simulink model "Matematico_Modelo_final"  (R2022b)
settings: Solver=VariableStepAuto  StartTime=0.0  StopTime=200  RelTol=1e-3
values from neighbouring files (symbols this model uses):
  B = 0.0244    [Datos_motor.m]
  Ff = 0.74    [Datos_motor.m]
  G = 50    [Datos_motor.m]
  J1 = 0.00072    [Datos_motor.m]
  J2 = 0.00072    [Datos_motor.m]
  Jg = 9.158    [Datos_motor.m]
  Jm = 9.158    [Datos_motor.m]
  K1 = 7.23e10    (= 72300000000)    [Datos_motor.m]
  K2 = 7.23e10    (= 72300000000)    [Datos_motor.m]
  K3 = 7.23e10    (= 72300000000)    [Datos_motor.m]
  Ke = 0.623    [Datos_motor.m]
  Kt = 0.333    [Datos_motor.m]
  L = 0.00163    [Datos_motor.m]
  Mcx = 1.1414    [Datos_motor.m]
  Mcy = 2.036    [Datos_motor.m]
  McZ = 0.839    [Datos_motor.m]
  R = 2.1    [Datos_motor.m]
  T = 2.059    [Datos_motor.m]
libraries: slpidlib x3
settings Model: Creator=aleal  LastModifiedBy=USER
settings DebuggingCC: UnconnectedInputMsg=warning  UnconnectedOutputMsg=warning  UnconnectedLineMsg=warning
settings ModelReferenceCC: EnableRefExpFcnMdlSchedulingChecks=on
settings RTWCC: DLArmComputeVersion=19.05

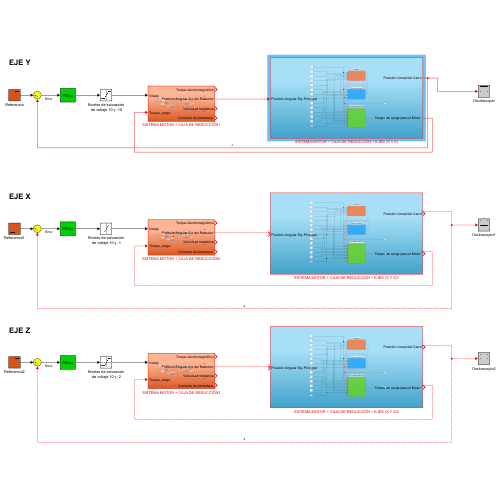
[thumbnail: Simulink's stored preview of the top-level diagram]
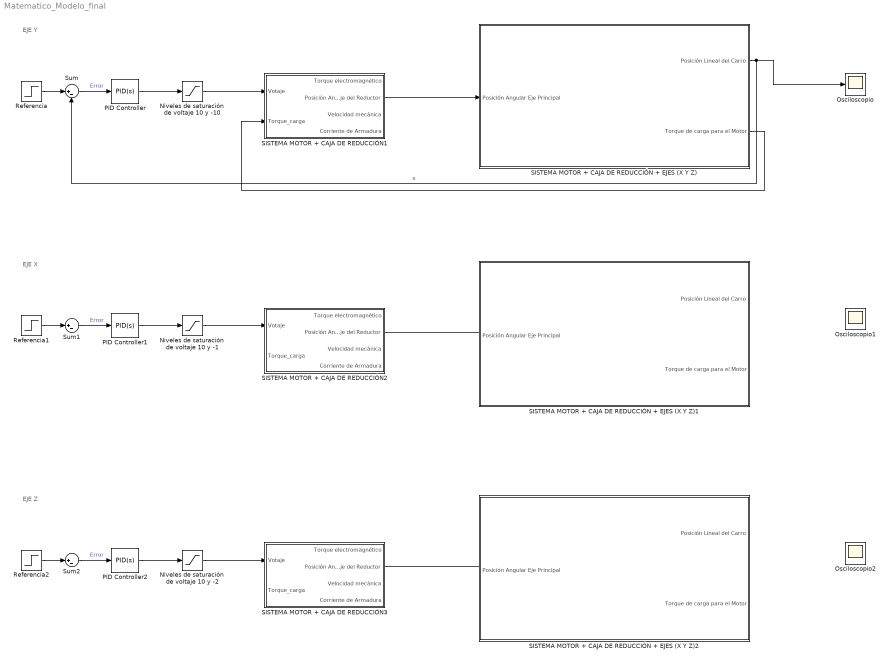
== system Matematico_Modelo_final ==
  note: EJE Z
  note: EJE Y
  note: EJE X
  Niveles de saturación de voltaje 10 y -1 : Saturate  UpperLimit=10  LowerLimit=-10
  Niveles de saturación de voltaje 10 y -10 : Saturate  UpperLimit=10  LowerLimit=-10
  Niveles de saturación de voltaje 10 y -2 : Saturate  UpperLimit=10  LowerLimit=-10
  Osciloscopio : Scope
  Osciloscopio1 : Scope
  Osciloscopio2 : Scope
  PID Controller : slpidlib/PID Controller  Controller=PID  Form=Parallel  TimeDomain=Continuous-time  UseExternalTs=off  SampleTime=-1  IntegratorMethod=Forward Euler  FilterMethod=Forward Euler  ControllerParametersSource=internal  P=10.0  I=1.0  UseKiTs=off  D=1.3  N=100  UseFilter=on  TunerSelectOption=Transfer Function Based (PID Tuner App)  InitialConditionSource=internal  InitialConditionForIntegrator=0  InitialConditionForFilter=0  DifferentiatorICPrevScaledInput=0  ExternalReset=none  TrackingMode=off  Kt=1  LimitOutput=off  SatLimitsSource=internal  UpperSaturationLimit=inf  LowerSaturationLimit=-inf  LinearizeAsGain=on  AntiWindupMode=none  Kb=1  LimitIntegrator=off  UpperIntegratorSaturationLimit=inf  LowerIntegratorSaturationLimit=-inf  POutMin=[]  POutMax=[]  IOutMin=[]  IOutMax=[]  DOutMin=[]  DOutMax=[]  NOutMin=[]  NOutMax=[]  SumOutMin=[]  SumOutMax=[]  SaturationOutMin=[]  SaturationOutMax=[]  PParamMin=[]  PParamMax=[]  IParamMin=[]  IParamMax=[]  DParamMin=[]  DParamMax=[]  NParamMin=[]  NParamMax=[]  KbParamMin=[]  KbParamMax=[]  KtParamMin=[]  KtParamMax=[]  KbOutMin=[]  KbOutMax=[]  KtOutMin=[]  KtOutMax=[]  IntegratorOutMin=[]  IntegratorOutMax=[]  FilterOutMin=[]  FilterOutMax=[]  SumI1OutMin=[]  SumI1OutMax=[]  SumI2OutMin=[]  SumI2OutMax=[]  SumI3OutMin=[]  SumI3OutMax=[]  SumI4OutMin=[]  SumI4OutMax=[]  SumDOutMin=[]  SumDOutMax=[]  DifferentiatorOutMin=[]  DifferentiatorOutMax=[]  FilterDiffOutCoefMin=[]  FilterDiffOutCoefMax=[]  ReciprocalOutMin=[]  ReciprocalOutMax=[]  SumDenOutMin=[]  SumDenOutMax=[]  SumNumOutMin=[]  SumNumOutMax=[]  DivideOutMin=[]  DivideOutMax=[]  UdiffTsProdOutMin=[]  UdiffTsProdOutMax=[]  NTsProdOutMin=[]  NTsProdOutMax=[]  UintegralTsProdOutMin=[]  UintegralTsProdOutMax=[]  UngainTsProdOutMin=[]  UngainTsProdOutMax=[]  ClampingZeroOutDataTypeStr=Inherit: Inherit via back propagation  ClampingZeroOutMin=[]  ClampingZeroOutMax=[]  FilterDenConstantOutDataTypeStr=Inherit: Inherit via back propagation  FilterDenConstantOutMin=[]  FilterDenConstantOutMax=[]  PCopyOutDataTypeStr=Inherit: Inherit via back propagation  PCopyOutMin=[]  PCopyOutMax=[]  NCopyOutDataTypeStr=Inherit: Inherit via back propagation  NCopyOutMin=[]  NCopyOutMax=[]  IntegratorContinuousStateAttributes=''  IntegratorStateMustResolveToSignalObject=off  IntegratorRTWStateStorageClass=Auto  FilterContinuousStateAttributes=''  FilterStateMustResolveToSignalObject=off  FilterRTWStateStorageClass=Auto  ParallelPVariant=InternalParameters  IdealPVariant=Disabled  IVariant=InternalParameters  DVariant=InternalParameters  IntegratorVariant=Continuous  SatVariant=Disabled  AWVariant=Passthrough  PCopyVariant=Disabled  TRVariant=Disabled  FdbkBlocksVariant=Forward  IdealPFdbkVariant=Disabled  SatFdbkVariant=Disabled  DerivativeFilterVariant=ContFilter  NVariant=InternalParameters  NCopyVariant=Disabled  FilterICVariant=InternalICsFilter  IntegratorICVariant=InternalICs  ExternalResetVariant=Disabled  TRSumVariant=Passthrough  SumFdbkVariant=Disabled  SumVariant=Sum_PID  TsampFilterVariant=InternalTs  TsampNgainVariant=Passthrough  TsampIntegralVariant=Passthrough  ExternalSaturationOutDataTypeStr=Inherit: Same as second input
  PID Controller1 : slpidlib/PID Controller  Controller=PID  Form=Parallel  TimeDomain=Continuous-time  UseExternalTs=off  SampleTime=-1  IntegratorMethod=Forward Euler  FilterMethod=Forward Euler  ControllerParametersSource=internal  P=9.0  I=0.7  UseKiTs=off  D=0.8  N=100  UseFilter=on  TunerSelectOption=Transfer Function Based (PID Tuner App)  InitialConditionSource=internal  InitialConditionForIntegrator=0  InitialConditionForFilter=0  DifferentiatorICPrevScaledInput=0  ExternalReset=none  TrackingMode=off  Kt=1  LimitOutput=off  SatLimitsSource=internal  UpperSaturationLimit=inf  LowerSaturationLimit=-inf  LinearizeAsGain=on  AntiWindupMode=none  Kb=1  LimitIntegrator=off  UpperIntegratorSaturationLimit=inf  LowerIntegratorSaturationLimit=-inf  POutMin=[]  POutMax=[]  IOutMin=[]  IOutMax=[]  DOutMin=[]  DOutMax=[]  NOutMin=[]  NOutMax=[]  SumOutMin=[]  SumOutMax=[]  SaturationOutMin=[]  SaturationOutMax=[]  PParamMin=[]  PParamMax=[]  IParamMin=[]  IParamMax=[]  DParamMin=[]  DParamMax=[]  NParamMin=[]  NParamMax=[]  KbParamMin=[]  KbParamMax=[]  KtParamMin=[]  KtParamMax=[]  KbOutMin=[]  KbOutMax=[]  KtOutMin=[]  KtOutMax=[]  IntegratorOutMin=[]  IntegratorOutMax=[]  FilterOutMin=[]  FilterOutMax=[]  SumI1OutMin=[]  SumI1OutMax=[]  SumI2OutMin=[]  SumI2OutMax=[]  SumI3OutMin=[]  SumI3OutMax=[]  SumI4OutMin=[]  SumI4OutMax=[]  SumDOutMin=[]  SumDOutMax=[]  DifferentiatorOutMin=[]  DifferentiatorOutMax=[]  FilterDiffOutCoefMin=[]  FilterDiffOutCoefMax=[]  ReciprocalOutMin=[]  ReciprocalOutMax=[]  SumDenOutMin=[]  SumDenOutMax=[]  SumNumOutMin=[]  SumNumOutMax=[]  DivideOutMin=[]  DivideOutMax=[]  UdiffTsProdOutMin=[]  UdiffTsProdOutMax=[]  NTsProdOutMin=[]  NTsProdOutMax=[]  UintegralTsProdOutMin=[]  UintegralTsProdOutMax=[]  UngainTsProdOutMin=[]  UngainTsProdOutMax=[]  ClampingZeroOutDataTypeStr=Inherit: Inherit via back propagation  ClampingZeroOutMin=[]  ClampingZeroOutMax=[]  FilterDenConstantOutDataTypeStr=Inherit: Inherit via back propagation  FilterDenConstantOutMin=[]  FilterDenConstantOutMax=[]  PCopyOutDataTypeStr=Inherit: Inherit via back propagation  PCopyOutMin=[]  PCopyOutMax=[]  NCopyOutDataTypeStr=Inherit: Inherit via back propagation  NCopyOutMin=[]  NCopyOutMax=[]  IntegratorContinuousStateAttributes=''  IntegratorStateMustResolveToSignalObject=off  IntegratorRTWStateStorageClass=Auto  FilterContinuousStateAttributes=''  FilterStateMustResolveToSignalObject=off  FilterRTWStateStorageClass=Auto  ParallelPVariant=InternalParameters  IdealPVariant=Disabled  IVariant=InternalParameters  DVariant=InternalParameters  IntegratorVariant=Continuous  SatVariant=Disabled  AWVariant=Passthrough  PCopyVariant=Disabled  TRVariant=Disabled  FdbkBlocksVariant=Forward  IdealPFdbkVariant=Disabled  SatFdbkVariant=Disabled  DerivativeFilterVariant=ContFilter  NVariant=InternalParameters  NCopyVariant=Disabled  FilterICVariant=InternalICsFilter  IntegratorICVariant=InternalICs  ExternalResetVariant=Disabled  TRSumVariant=Passthrough  SumFdbkVariant=Disabled  SumVariant=Sum_PID  TsampFilterVariant=InternalTs  TsampNgainVariant=Passthrough  TsampIntegralVariant=Passthrough  ExternalSaturationOutDataTypeStr=Inherit: Same as second input
  PID Controller2 : slpidlib/PID Controller  Controller=PID  Form=Parallel  TimeDomain=Continuous-time  UseExternalTs=off  SampleTime=-1  IntegratorMethod=Forward Euler  FilterMethod=Forward Euler  ControllerParametersSource=internal  P=9.0  I=0.5  UseKiTs=off  D=0.4  N=100  UseFilter=on  TunerSelectOption=Transfer Function Based (PID Tuner App)  InitialConditionSource=internal  InitialConditionForIntegrator=0  InitialConditionForFilter=0  DifferentiatorICPrevScaledInput=0  ExternalReset=none  TrackingMode=off  Kt=1  LimitOutput=off  SatLimitsSource=internal  UpperSaturationLimit=inf  LowerSaturationLimit=-inf  LinearizeAsGain=on  AntiWindupMode=none  Kb=1  LimitIntegrator=off  UpperIntegratorSaturationLimit=inf  LowerIntegratorSaturationLimit=-inf  POutMin=[]  POutMax=[]  IOutMin=[]  IOutMax=[]  DOutMin=[]  DOutMax=[]  NOutMin=[]  NOutMax=[]  SumOutMin=[]  SumOutMax=[]  SaturationOutMin=[]  SaturationOutMax=[]  PParamMin=[]  PParamMax=[]  IParamMin=[]  IParamMax=[]  DParamMin=[]  DParamMax=[]  NParamMin=[]  NParamMax=[]  KbParamMin=[]  KbParamMax=[]  KtParamMin=[]  KtParamMax=[]  KbOutMin=[]  KbOutMax=[]  KtOutMin=[]  KtOutMax=[]  IntegratorOutMin=[]  IntegratorOutMax=[]  FilterOutMin=[]  FilterOutMax=[]  SumI1OutMin=[]  SumI1OutMax=[]  SumI2OutMin=[]  SumI2OutMax=[]  SumI3OutMin=[]  SumI3OutMax=[]  SumI4OutMin=[]  SumI4OutMax=[]  SumDOutMin=[]  SumDOutMax=[]  DifferentiatorOutMin=[]  DifferentiatorOutMax=[]  FilterDiffOutCoefMin=[]  FilterDiffOutCoefMax=[]  ReciprocalOutMin=[]  ReciprocalOutMax=[]  SumDenOutMin=[]  SumDenOutMax=[]  SumNumOutMin=[]  SumNumOutMax=[]  DivideOutMin=[]  DivideOutMax=[]  UdiffTsProdOutMin=[]  UdiffTsProdOutMax=[]  NTsProdOutMin=[]  NTsProdOutMax=[]  UintegralTsProdOutMin=[]  UintegralTsProdOutMax=[]  UngainTsProdOutMin=[]  UngainTsProdOutMax=[]  ClampingZeroOutDataTypeStr=Inherit: Inherit via back propagation  ClampingZeroOutMin=[]  ClampingZeroOutMax=[]  FilterDenConstantOutDataTypeStr=Inherit: Inherit via back propagation  FilterDenConstantOutMin=[]  FilterDenConstantOutMax=[]  PCopyOutDataTypeStr=Inherit: Inherit via back propagation  PCopyOutMin=[]  PCopyOutMax=[]  NCopyOutDataTypeStr=Inherit: Inherit via back propagation  NCopyOutMin=[]  NCopyOutMax=[]  IntegratorContinuousStateAttributes=''  IntegratorStateMustResolveToSignalObject=off  IntegratorRTWStateStorageClass=Auto  FilterContinuousStateAttributes=''  FilterStateMustResolveToSignalObject=off  FilterRTWStateStorageClass=Auto  ParallelPVariant=InternalParameters  IdealPVariant=Disabled  IVariant=InternalParameters  DVariant=InternalParameters  IntegratorVariant=Continuous  SatVariant=Disabled  AWVariant=Passthrough  PCopyVariant=Disabled  TRVariant=Disabled  FdbkBlocksVariant=Forward  IdealPFdbkVariant=Disabled  SatFdbkVariant=Disabled  DerivativeFilterVariant=ContFilter  NVariant=InternalParameters  NCopyVariant=Disabled  FilterICVariant=InternalICsFilter  IntegratorICVariant=InternalICs  ExternalResetVariant=Disabled  TRSumVariant=Passthrough  SumFdbkVariant=Disabled  SumVariant=Sum_PID  TsampFilterVariant=InternalTs  TsampNgainVariant=Passthrough  TsampIntegralVariant=Passthrough  ExternalSaturationOutDataTypeStr=Inherit: Same as second input
  Referencia : Step  After=0.15  SampleTime=0
  Referencia1 : Step  After=0.15  SampleTime=0
  Referencia2 : Step  After=0.15  SampleTime=0
  SISTEMA MOTOR + CAJA DE REDUCCIÓN + EJES (X Y Z) : Subsystem
  SISTEMA MOTOR + CAJA DE REDUCCIÓN + EJES (X Y Z)1 : Subsystem
  SISTEMA MOTOR + CAJA DE REDUCCIÓN + EJES (X Y Z)2 : Subsystem
  SISTEMA MOTOR + CAJA DE REDUCCIÓN1 : Subsystem
  SISTEMA MOTOR + CAJA DE REDUCCIÓN2 : Subsystem
  SISTEMA MOTOR + CAJA DE REDUCCIÓN3 : Subsystem
  Sum : Sum  Inputs=|+-
  Sum1 : Sum  Inputs=|+-
  Sum2 : Sum  Inputs=|+-
  wires:
  SISTEMA MOTOR + CAJA DE REDUCCIÓN1/2(Posición Angular Eje del Reductor) -> SISTEMA MOTOR + CAJA DE REDUCCIÓN + EJES (X Y Z)/1("Posición Angular Eje Principal ")
  SISTEMA MOTOR + CAJA DE REDUCCIÓN + EJES (X Y Z)/2("Torque de carga para el Motor ") -> SISTEMA MOTOR + CAJA DE REDUCCIÓN1/2("Torque_carga ")
  Niveles de saturación de voltaje 10 y -10/1 -> SISTEMA MOTOR + CAJA DE REDUCCIÓN1/1(Votaje)
  SISTEMA MOTOR + CAJA DE REDUCCIÓN + EJES (X Y Z)/1(Posición Lineal del Carro) -> Sum/2, Osciloscopio/1  "x"
  PID Controller/1 -> Niveles de saturación de voltaje 10 y -10/1
  Sum/1 -> PID Controller/1  "Error"
  Referencia/1 -> Sum/1
  ? -> Sum1/2, Osciloscopio1/1  "x"
  Niveles de saturación de voltaje 10 y -1/1 -> SISTEMA MOTOR + CAJA DE REDUCCIÓN2/1(Votaje)
  Referencia1/1 -> Sum1/1
  PID Controller1/1 -> Niveles de saturación de voltaje 10 y -1/1
  ? -> SISTEMA MOTOR + CAJA DE REDUCCIÓN2/2("Torque_carga ")
  Sum1/1 -> PID Controller1/1  "Error"
  SISTEMA MOTOR + CAJA DE REDUCCIÓN2/2(Posición Angular Eje del Reductor) -> ?
  ? -> Sum2/2, Osciloscopio2/1  "x"
  Niveles de saturación de voltaje 10 y -2/1 -> SISTEMA MOTOR + CAJA DE REDUCCIÓN3/1(Votaje)
  Referencia2/1 -> Sum2/1
  PID Controller2/1 -> Niveles de saturación de voltaje 10 y -2/1
  ? -> SISTEMA MOTOR + CAJA DE REDUCCIÓN3/2("Torque_carga ")
  Sum2/1 -> PID Controller2/1  "Error"
  SISTEMA MOTOR + CAJA DE REDUCCIÓN3/2(Posición Angular Eje del Reductor) -> ?

== system Matematico_Modelo_final/SISTEMA MOTOR + CAJA DE REDUCCIÓN + EJES (X Y Z) ==
  note: CARRO
  note: POLEA FINAL
  note: POLEA DE MOTOR
  "Posición Angular Eje Principal " : Inport
  Caja de reducción : Constant  Value=G
  Coeficiente de eleasticidad de la polea 1 : Constant  Value=K1
  Coeficiente de eleasticidad de la polea 2 : Constant  Value=K2
  Coeficiente de eleasticidad de la polea 3 : Constant  Value=K3
  Constante 1 : Constant
  Fricción de carrito : Constant  Value=Ff
  Inercia caja de reducción 1 : Constant  Value=Jg
  Inercia caja de reducción 2 : Constant  Value=Jm
  Inercia polea 1 : Constant  Value=J1
  Inercia polea 2 : Constant  Value=J2
  Masa carrito : Constant  Value=Mcy
  Radio de la polea : Constant  Value=R
  Torque de motor : Constant  Value=T
  q1''=[G.T-R.(K1.(R.q1-X)-K3.(R.q2-Rq1))] J1+G^2.(Jg+Jm) : Subsystem
  q2´´=R[K2.(X-R.q2)-K3.(R.q2-q1)] J2 : Subsystem
  x´´=([K1.(R.q1-X)-K2.(X-R.q2)]-Ff) MC : Subsystem
  Posición Lineal del Carro : Outport
  "Torque de carga para el Motor " : Outport  Port=2
  wires:
  Constante 1/1 -> q2´´=R[K2.(X-R.q2)-K3.(R.q2-q1)] J2/1(Constante 1), q1''=[G.T-R.(K1.(R.q1-X)-K3.(R.q2-Rq1))] J1+G^2.(Jg+Jm)/1(Constante 1), x´´=([K1.(R.q1-X)-K2.(X-R.q2)]-Ff) MC/1(Constante 1)
  Masa carrito/1 -> x´´=([K1.(R.q1-X)-K2.(X-R.q2)]-Ff) MC/2("Mc ")
  Fricción de carrito/1 -> x´´=([K1.(R.q1-X)-K2.(X-R.q2)]-Ff) MC/3(Ff)
  Coeficiente de eleasticidad de la polea 1/1 -> x´´=([K1.(R.q1-X)-K2.(X-R.q2)]-Ff) MC/4(K1), q1''=[G.T-R.(K1.(R.q1-X)-K3.(R.q2-Rq1))] J1+G^2.(Jg+Jm)/2("K1 ")
  Radio de la polea/1 -> q1''=[G.T-R.(K1.(R.q1-X)-K3.(R.q2-Rq1))] J1+G^2.(Jg+Jm)/8(R), x´´=([K1.(R.q1-X)-K2.(X-R.q2)]-Ff) MC/5(R), q2´´=R[K2.(X-R.q2)-K3.(R.q2-q1)] J2/4(R)
  Coeficiente de eleasticidad de la polea 2/1 -> x´´=([K1.(R.q1-X)-K2.(X-R.q2)]-Ff) MC/6(K2), q2´´=R[K2.(X-R.q2)-K3.(R.q2-q1)] J2/5(K2)
  Inercia polea 2/1 -> q2´´=R[K2.(X-R.q2)-K3.(R.q2-q1)] J2/2("J2 ")
  Coeficiente de eleasticidad de la polea 3/1 -> q1''=[G.T-R.(K1.(R.q1-X)-K3.(R.q2-Rq1))] J1+G^2.(Jg+Jm)/9(K3), q2´´=R[K2.(X-R.q2)-K3.(R.q2-q1)] J2/3(K3)
  q2´´=R[K2.(X-R.q2)-K3.(R.q2-q1)] J2/1(q2) -> q1''=[G.T-R.(K1.(R.q1-X)-K3.(R.q2-Rq1))] J1+G^2.(Jg+Jm)/11(q2), x´´=([K1.(R.q1-X)-K2.(X-R.q2)]-Ff) MC/7(" q2")
  Inercia polea 1/1 -> q1''=[G.T-R.(K1.(R.q1-X)-K3.(R.q2-Rq1))] J1+G^2.(Jg+Jm)/3(J1)
  Caja de reducción/1 -> q1''=[G.T-R.(K1.(R.q1-X)-K3.(R.q2-Rq1))] J1+G^2.(Jg+Jm)/4(G)
  Inercia caja de reducción 1/1 -> q1''=[G.T-R.(K1.(R.q1-X)-K3.(R.q2-Rq1))] J1+G^2.(Jg+Jm)/5(Jg)
  Inercia caja de reducción 2/1 -> q1''=[G.T-R.(K1.(R.q1-X)-K3.(R.q2-Rq1))] J1+G^2.(Jg+Jm)/6(Jm)
  Torque de motor/1 -> q1''=[G.T-R.(K1.(R.q1-X)-K3.(R.q2-Rq1))] J1+G^2.(Jg+Jm)/7(T)
  "Posición Angular Eje Principal "/1 -> x´´=([K1.(R.q1-X)-K2.(X-R.q2)]-Ff) MC/8(q1), q2´´=R[K2.(X-R.q2)-K3.(R.q2-q1)] J2/7(q1), q1''=[G.T-R.(K1.(R.q1-X)-K3.(R.q2-Rq1))] J1+G^2.(Jg+Jm)/10(q1)  "q1"
  q1''=[G.T-R.(K1.(R.q1-X)-K3.(R.q2-Rq1))] J1+G^2.(Jg+Jm)/1("TL ") -> "Torque de carga para el Motor "/1
  x´´=([K1.(R.q1-X)-K2.(X-R.q2)]-Ff) MC/1(X) -> q2´´=R[K2.(X-R.q2)-K3.(R.q2-q1)] J2/6(x), Posición Lineal del Carro/1, q1''=[G.T-R.(K1.(R.q1-X)-K3.(R.q2-Rq1))] J1+G^2.(Jg+Jm)/12(X)

== system Matematico_Modelo_final/SISTEMA MOTOR + CAJA DE REDUCCIÓN + EJES (X Y Z)1 ==
  note: POLEA DE MOTOR
  note: CARRO
  note: POLEA FINAL
  "Posición Angular Eje Principal " : Inport
  Caja de reducción : Constant  Value=G
  Coeficiente de eleasticidad de la polea 1 : Constant  Value=K1
  Coeficiente de eleasticidad de la polea 2 : Constant  Value=K2
  Coeficiente de eleasticidad de la polea 3 : Constant  Value=K3
  Constante 1 : Constant
  Fricción de carrito : Constant  Value=Ff
  Inercia caja de reducción 1 : Constant  Value=Jg
  Inercia caja de reducción 2 : Constant  Value=Jm
  Inercia polea 1 : Constant  Value=J1
  Inercia polea 2 : Constant  Value=J2
  Masa carrito : Constant  Value=Mcx
  Radio de la polea : Constant  Value=R
  Torque de motor : Constant  Value=T
  q1''=[G.T-R.(K1.(R.q1-X)-K3.(R.q2-Rq1))] J1+G^2.(Jg+Jm) : Subsystem
  q2´´=R[K2.(X-R.q2)-K3.(R.q2-q1)] J2 : Subsystem
  x´´=([K1.(R.q1-X)-K2.(X-R.q2)]-Ff) MC : Subsystem
  Posición Lineal del Carro : Outport
  "Torque de carga para el Motor " : Outport  Port=2
  wires:
  Torque de motor/1 -> q1''=[G.T-R.(K1.(R.q1-X)-K3.(R.q2-Rq1))] J1+G^2.(Jg+Jm)/7(T)
  "Posición Angular Eje Principal "/1 -> x´´=([K1.(R.q1-X)-K2.(X-R.q2)]-Ff) MC/8(q1), q2´´=R[K2.(X-R.q2)-K3.(R.q2-q1)] J2/7(q1), q1''=[G.T-R.(K1.(R.q1-X)-K3.(R.q2-Rq1))] J1+G^2.(Jg+Jm)/10(q1)  "q1"
  q2´´=R[K2.(X-R.q2)-K3.(R.q2-q1)] J2/1(q2) -> q1''=[G.T-R.(K1.(R.q1-X)-K3.(R.q2-Rq1))] J1+G^2.(Jg+Jm)/11(q2), x´´=([K1.(R.q1-X)-K2.(X-R.q2)]-Ff) MC/7(" q2")
  Fricción de carrito/1 -> x´´=([K1.(R.q1-X)-K2.(X-R.q2)]-Ff) MC/3(Ff)
  Coeficiente de eleasticidad de la polea 1/1 -> x´´=([K1.(R.q1-X)-K2.(X-R.q2)]-Ff) MC/4(K1), q1''=[G.T-R.(K1.(R.q1-X)-K3.(R.q2-Rq1))] J1+G^2.(Jg+Jm)/2("K1 ")
  Coeficiente de eleasticidad de la polea 2/1 -> x´´=([K1.(R.q1-X)-K2.(X-R.q2)]-Ff) MC/6(K2), q2´´=R[K2.(X-R.q2)-K3.(R.q2-q1)] J2/5(K2)
  Inercia polea 2/1 -> q2´´=R[K2.(X-R.q2)-K3.(R.q2-q1)] J2/2("J2 ")
  Radio de la polea/1 -> q1''=[G.T-R.(K1.(R.q1-X)-K3.(R.q2-Rq1))] J1+G^2.(Jg+Jm)/8(R), x´´=([K1.(R.q1-X)-K2.(X-R.q2)]-Ff) MC/5(R), q2´´=R[K2.(X-R.q2)-K3.(R.q2-q1)] J2/4(R)
  Coeficiente de eleasticidad de la polea 3/1 -> q1''=[G.T-R.(K1.(R.q1-X)-K3.(R.q2-Rq1))] J1+G^2.(Jg+Jm)/9(K3), q2´´=R[K2.(X-R.q2)-K3.(R.q2-q1)] J2/3(K3)
  x´´=([K1.(R.q1-X)-K2.(X-R.q2)]-Ff) MC/1(X) -> q2´´=R[K2.(X-R.q2)-K3.(R.q2-q1)] J2/6(x), Posición Lineal del Carro/1, q1''=[G.T-R.(K1.(R.q1-X)-K3.(R.q2-Rq1))] J1+G^2.(Jg+Jm)/12(X)
  Inercia polea 1/1 -> q1''=[G.T-R.(K1.(R.q1-X)-K3.(R.q2-Rq1))] J1+G^2.(Jg+Jm)/3(J1)
  Inercia caja de reducción 1/1 -> q1''=[G.T-R.(K1.(R.q1-X)-K3.(R.q2-Rq1))] J1+G^2.(Jg+Jm)/5(Jg)
  Inercia caja de reducción 2/1 -> q1''=[G.T-R.(K1.(R.q1-X)-K3.(R.q2-Rq1))] J1+G^2.(Jg+Jm)/6(Jm)
  Caja de reducción/1 -> q1''=[G.T-R.(K1.(R.q1-X)-K3.(R.q2-Rq1))] J1+G^2.(Jg+Jm)/4(G)
  Masa carrito/1 -> x´´=([K1.(R.q1-X)-K2.(X-R.q2)]-Ff) MC/2("Mc ")
  q1''=[G.T-R.(K1.(R.q1-X)-K3.(R.q2-Rq1))] J1+G^2.(Jg+Jm)/1("TL ") -> "Torque de carga para el Motor "/1
  Constante 1/1 -> q2´´=R[K2.(X-R.q2)-K3.(R.q2-q1)] J2/1(Constante 1), q1''=[G.T-R.(K1.(R.q1-X)-K3.(R.q2-Rq1))] J1+G^2.(Jg+Jm)/1(Constante 1), x´´=([K1.(R.q1-X)-K2.(X-R.q2)]-Ff) MC/1(Constante 1)

== system Matematico_Modelo_final/SISTEMA MOTOR + CAJA DE REDUCCIÓN + EJES (X Y Z)2 ==
  note: POLEA DE MOTOR
  note: CARRO
  note: POLEA FINAL
  "Posición Angular Eje Principal " : Inport
  Caja de reducción : Constant  Value=G
  Coeficiente de eleasticidad de la polea 1 : Constant  Value=K1
  Coeficiente de eleasticidad de la polea 2 : Constant  Value=K2
  Coeficiente de eleasticidad de la polea 3 : Constant  Value=K3
  Constante 1 : Constant
  Fricción de carrito : Constant  Value=Ff
  Inercia caja de reducción 1 : Constant  Value=Jg
  Inercia caja de reducción 2 : Constant  Value=Jm
  Inercia polea 1 : Constant  Value=J1
  Inercia polea 2 : Constant  Value=J2
  Masa carrito : Constant  Value=McZ
  Radio de la polea : Constant  Value=R
  Torque de motor : Constant  Value=T
  q1''=[G.T-R.(K1.(R.q1-X)-K3.(R.q2-Rq1))] J1+G^2.(Jg+Jm) : Subsystem
  q2´´=R[K2.(X-R.q2)-K3.(R.q2-q1)] J2 : Subsystem
  x´´=([K1.(R.q1-X)-K2.(X-R.q2)]-Ff) MC : Subsystem
  Posición Lineal del Carro : Outport
  "Torque de carga para el Motor " : Outport  Port=2
  wires:
  Torque de motor/1 -> q1''=[G.T-R.(K1.(R.q1-X)-K3.(R.q2-Rq1))] J1+G^2.(Jg+Jm)/7(T)
  "Posición Angular Eje Principal "/1 -> x´´=([K1.(R.q1-X)-K2.(X-R.q2)]-Ff) MC/8(q1), q2´´=R[K2.(X-R.q2)-K3.(R.q2-q1)] J2/7(q1), q1''=[G.T-R.(K1.(R.q1-X)-K3.(R.q2-Rq1))] J1+G^2.(Jg+Jm)/10(q1)  "q1"
  q2´´=R[K2.(X-R.q2)-K3.(R.q2-q1)] J2/1(q2) -> q1''=[G.T-R.(K1.(R.q1-X)-K3.(R.q2-Rq1))] J1+G^2.(Jg+Jm)/11(q2), x´´=([K1.(R.q1-X)-K2.(X-R.q2)]-Ff) MC/7(" q2")
  Fricción de carrito/1 -> x´´=([K1.(R.q1-X)-K2.(X-R.q2)]-Ff) MC/3(Ff)
  Coeficiente de eleasticidad de la polea 1/1 -> x´´=([K1.(R.q1-X)-K2.(X-R.q2)]-Ff) MC/4(K1), q1''=[G.T-R.(K1.(R.q1-X)-K3.(R.q2-Rq1))] J1+G^2.(Jg+Jm)/2("K1 ")
  Coeficiente de eleasticidad de la polea 2/1 -> x´´=([K1.(R.q1-X)-K2.(X-R.q2)]-Ff) MC/6(K2), q2´´=R[K2.(X-R.q2)-K3.(R.q2-q1)] J2/5(K2)
  Inercia polea 2/1 -> q2´´=R[K2.(X-R.q2)-K3.(R.q2-q1)] J2/2("J2 ")
  Radio de la polea/1 -> q1''=[G.T-R.(K1.(R.q1-X)-K3.(R.q2-Rq1))] J1+G^2.(Jg+Jm)/8(R), x´´=([K1.(R.q1-X)-K2.(X-R.q2)]-Ff) MC/5(R), q2´´=R[K2.(X-R.q2)-K3.(R.q2-q1)] J2/4(R)
  Coeficiente de eleasticidad de la polea 3/1 -> q1''=[G.T-R.(K1.(R.q1-X)-K3.(R.q2-Rq1))] J1+G^2.(Jg+Jm)/9(K3), q2´´=R[K2.(X-R.q2)-K3.(R.q2-q1)] J2/3(K3)
  x´´=([K1.(R.q1-X)-K2.(X-R.q2)]-Ff) MC/1(X) -> q2´´=R[K2.(X-R.q2)-K3.(R.q2-q1)] J2/6(x), Posición Lineal del Carro/1, q1''=[G.T-R.(K1.(R.q1-X)-K3.(R.q2-Rq1))] J1+G^2.(Jg+Jm)/12(X)
  Inercia polea 1/1 -> q1''=[G.T-R.(K1.(R.q1-X)-K3.(R.q2-Rq1))] J1+G^2.(Jg+Jm)/3(J1)
  Inercia caja de reducción 1/1 -> q1''=[G.T-R.(K1.(R.q1-X)-K3.(R.q2-Rq1))] J1+G^2.(Jg+Jm)/5(Jg)
  Inercia caja de reducción 2/1 -> q1''=[G.T-R.(K1.(R.q1-X)-K3.(R.q2-Rq1))] J1+G^2.(Jg+Jm)/6(Jm)
  Caja de reducción/1 -> q1''=[G.T-R.(K1.(R.q1-X)-K3.(R.q2-Rq1))] J1+G^2.(Jg+Jm)/4(G)
  Masa carrito/1 -> x´´=([K1.(R.q1-X)-K2.(X-R.q2)]-Ff) MC/2("Mc ")
  q1''=[G.T-R.(K1.(R.q1-X)-K3.(R.q2-Rq1))] J1+G^2.(Jg+Jm)/1("TL ") -> "Torque de carga para el Motor "/1
  Constante 1/1 -> q2´´=R[K2.(X-R.q2)-K3.(R.q2-q1)] J2/1(Constante 1), q1''=[G.T-R.(K1.(R.q1-X)-K3.(R.q2-Rq1))] J1+G^2.(Jg+Jm)/1(Constante 1), x´´=([K1.(R.q1-X)-K2.(X-R.q2)]-Ff) MC/1(Constante 1)

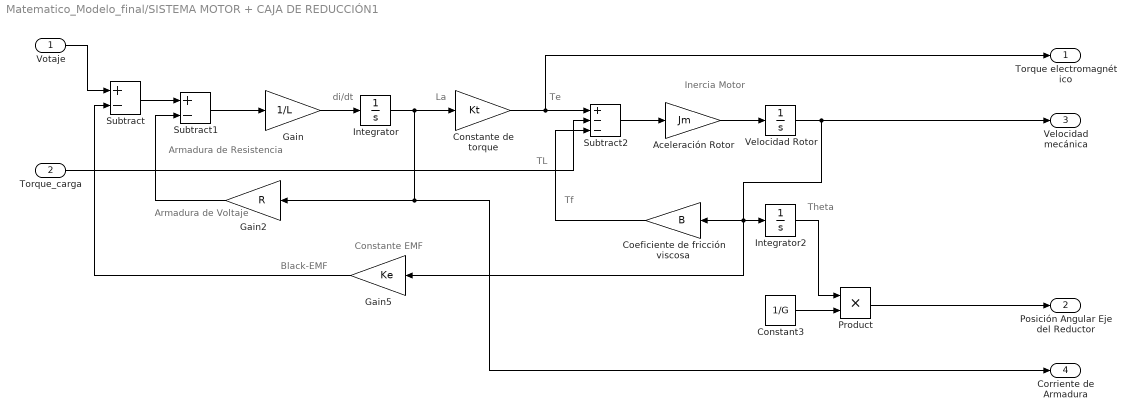
== system Matematico_Modelo_final/SISTEMA MOTOR + CAJA DE REDUCCIÓN1 ==
  note: Black-EMF
  note: Armadura de
      | Resistencia
  note: TL
  note: Tf
  note: Armadura de
      | Voltaje
  note: Te
  note: La
  note: Constante EMF
  note: di/dt
  note: Theta
  note: Inercia Motor
  Votaje : Inport
  "Torque_carga " : Inport  Port=2
  Aceleración Rotor : Gain  Gain=Jm
  Coeficiente de fricción viscosa : Gain  Gain=B
  Constant3 : Constant  Value=1/G
  Constante de torque : Gain  Gain=Kt
  Gain : Gain  Gain=1/L
  Gain2 : Gain  Gain=R
  Gain5 : Gain  Gain=Ke
  Integrator : Integrator
  Integrator2 : Integrator
  Product : Product
  Subtract : Sum  Inputs=+-
  Subtract1 : Sum  Inputs=+-
  Subtract2 : Sum  Inputs=+--
  Velocidad Rotor : Integrator
  Torque electromagnético : Outport  VectorParamsAs1DForOutWhenUnconnected=off
  Posición Angular Eje del Reductor : Outport  Port=2  VectorParamsAs1DForOutWhenUnconnected=off
  Velocidad mecánica : Outport  Port=3  VectorParamsAs1DForOutWhenUnconnected=off
  "Corriente de Armadura " : Outport  Port=4  VectorParamsAs1DForOutWhenUnconnected=off
  wires:
  Gain/1 -> Integrator/1
  Subtract/1 -> Subtract1/1
  Constante de torque/1 -> Torque electromagnético/1, Subtract2/1
  Subtract2/1 -> Aceleración Rotor/1
  Coeficiente de fricción viscosa/1 -> Subtract2/3
  Integrator/1 -> "Corriente de Armadura "/1, Gain2/1, Constante de torque/1
  Gain5/1 -> Subtract/2
  Subtract1/1 -> Gain/1
  Velocidad Rotor/1 -> Gain5/1, Coeficiente de fricción viscosa/1, Integrator2/1, Velocidad mecánica/1
  Aceleración Rotor/1 -> Velocidad Rotor/1
  "Torque_carga "/1 -> Subtract2/2
  Votaje/1 -> Subtract/1
  Gain2/1 -> Subtract1/2
  Product/1 -> Posición Angular Eje del Reductor/1
  Constant3/1 -> Product/2
  Integrator2/1 -> Product/1

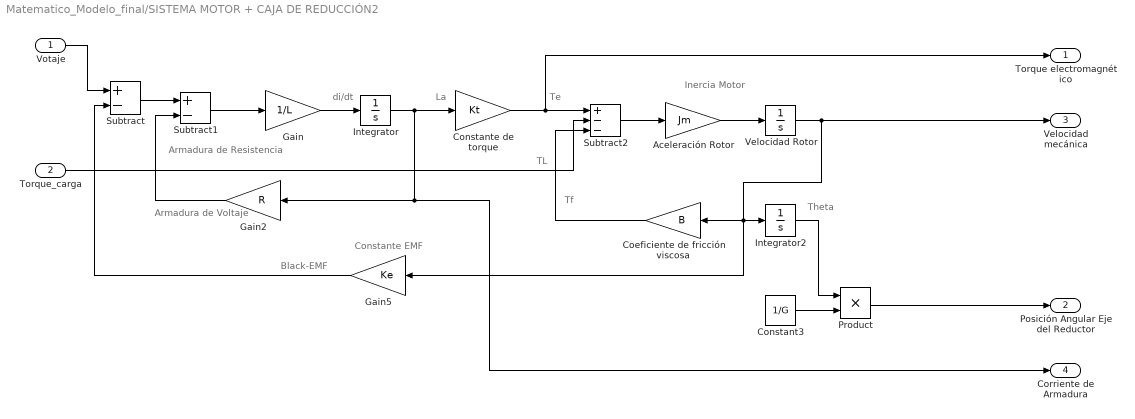
== system Matematico_Modelo_final/SISTEMA MOTOR + CAJA DE REDUCCIÓN2 ==
  note: Black-EMF
  note: Armadura de
      | Resistencia
  note: TL
  note: Tf
  note: Armadura de
      | Voltaje
  note: Te
  note: La
  note: Constante EMF
  note: di/dt
  note: Theta
  note: Inercia Motor
  Votaje : Inport
  "Torque_carga " : Inport  Port=2
  Aceleración Rotor : Gain  Gain=Jm
  Coeficiente de fricción viscosa : Gain  Gain=B
  Constant3 : Constant  Value=1/G
  Constante de torque : Gain  Gain=Kt
  Gain : Gain  Gain=1/L
  Gain2 : Gain  Gain=R
  Gain5 : Gain  Gain=Ke
  Integrator : Integrator
  Integrator2 : Integrator
  Product : Product
  Subtract : Sum  Inputs=+-
  Subtract1 : Sum  Inputs=+-
  Subtract2 : Sum  Inputs=+--
  Velocidad Rotor : Integrator
  Torque electromagnético : Outport  VectorParamsAs1DForOutWhenUnconnected=off
  Posición Angular Eje del Reductor : Outport  Port=2  VectorParamsAs1DForOutWhenUnconnected=off
  Velocidad mecánica : Outport  Port=3  VectorParamsAs1DForOutWhenUnconnected=off
  "Corriente de Armadura " : Outport  Port=4  VectorParamsAs1DForOutWhenUnconnected=off
  wires:
  Gain/1 -> Integrator/1
  Subtract/1 -> Subtract1/1
  Constante de torque/1 -> Torque electromagnético/1, Subtract2/1
  Subtract2/1 -> Aceleración Rotor/1
  Coeficiente de fricción viscosa/1 -> Subtract2/3
  Integrator/1 -> "Corriente de Armadura "/1, Gain2/1, Constante de torque/1
  Gain5/1 -> Subtract/2
  Subtract1/1 -> Gain/1
  Velocidad Rotor/1 -> Gain5/1, Coeficiente de fricción viscosa/1, Integrator2/1, Velocidad mecánica/1
  Aceleración Rotor/1 -> Velocidad Rotor/1
  "Torque_carga "/1 -> Subtract2/2
  Votaje/1 -> Subtract/1
  Gain2/1 -> Subtract1/2
  Product/1 -> Posición Angular Eje del Reductor/1
  Constant3/1 -> Product/2
  Integrator2/1 -> Product/1

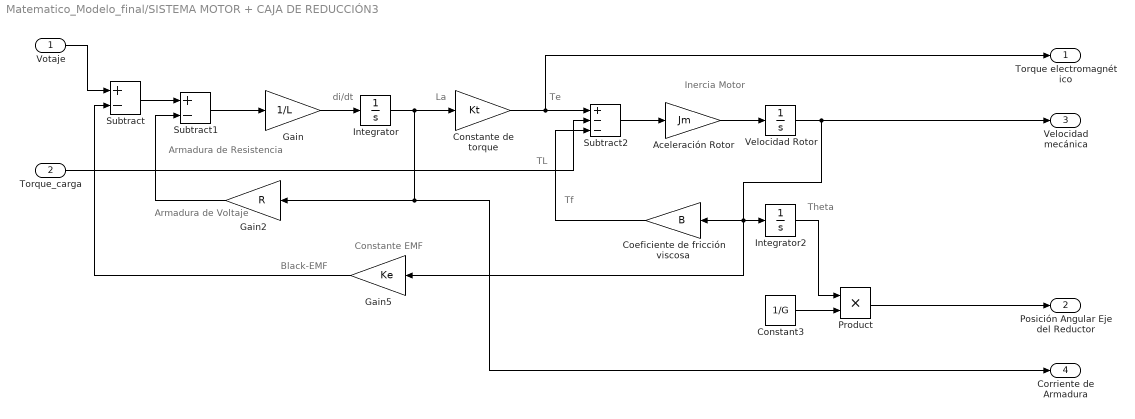
== system Matematico_Modelo_final/SISTEMA MOTOR + CAJA DE REDUCCIÓN3 ==
  note: Black-EMF
  note: Armadura de
      | Resistencia
  note: TL
  note: Tf
  note: Armadura de
      | Voltaje
  note: Te
  note: La
  note: Constante EMF
  note: di/dt
  note: Theta
  note: Inercia Motor
  Votaje : Inport
  "Torque_carga " : Inport  Port=2
  Aceleración Rotor : Gain  Gain=Jm
  Coeficiente de fricción viscosa : Gain  Gain=B
  Constant3 : Constant  Value=1/G
  Constante de torque : Gain  Gain=Kt
  Gain : Gain  Gain=1/L
  Gain2 : Gain  Gain=R
  Gain5 : Gain  Gain=Ke
  Integrator : Integrator
  Integrator2 : Integrator
  Product : Product
  Subtract : Sum  Inputs=+-
  Subtract1 : Sum  Inputs=+-
  Subtract2 : Sum  Inputs=+--
  Velocidad Rotor : Integrator
  Torque electromagnético : Outport  VectorParamsAs1DForOutWhenUnconnected=off
  Posición Angular Eje del Reductor : Outport  Port=2  VectorParamsAs1DForOutWhenUnconnected=off
  Velocidad mecánica : Outport  Port=3  VectorParamsAs1DForOutWhenUnconnected=off
  "Corriente de Armadura " : Outport  Port=4  VectorParamsAs1DForOutWhenUnconnected=off
  wires:
  Gain/1 -> Integrator/1
  Subtract/1 -> Subtract1/1
  Constante de torque/1 -> Torque electromagnético/1, Subtract2/1
  Subtract2/1 -> Aceleración Rotor/1
  Coeficiente de fricción viscosa/1 -> Subtract2/3
  Integrator/1 -> "Corriente de Armadura "/1, Gain2/1, Constante de torque/1
  Gain5/1 -> Subtract/2
  Subtract1/1 -> Gain/1
  Velocidad Rotor/1 -> Gain5/1, Coeficiente de fricción viscosa/1, Integrator2/1, Velocidad mecánica/1
  Aceleración Rotor/1 -> Velocidad Rotor/1
  "Torque_carga "/1 -> Subtract2/2
  Votaje/1 -> Subtract/1
  Gain2/1 -> Subtract1/2
  Product/1 -> Posición Angular Eje del Reductor/1
  Constant3/1 -> Product/2
  Integrator2/1 -> Product/1

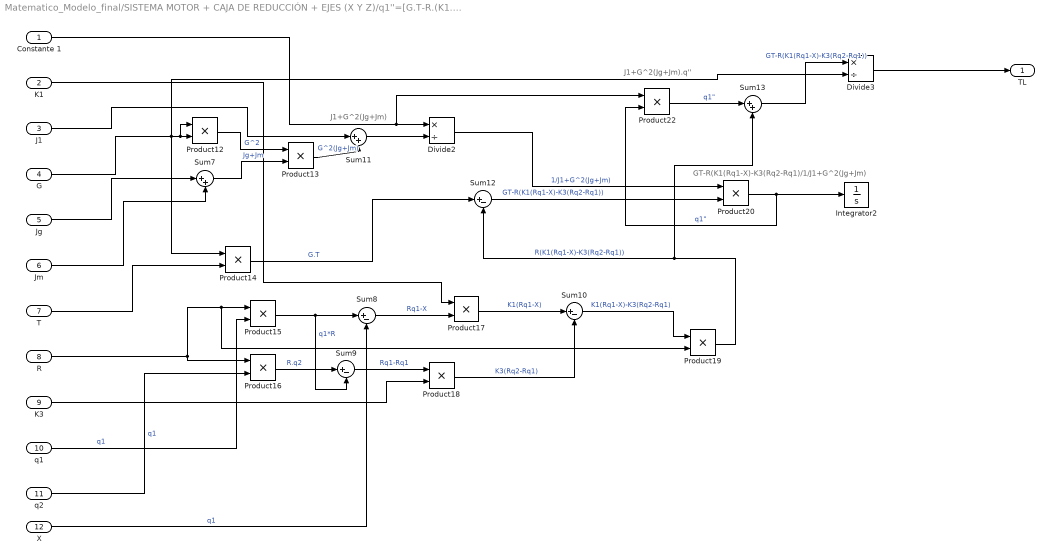
== system Matematico_Modelo_final/SISTEMA MOTOR + CAJA DE REDUCCIÓN + EJES (X Y Z)/q1''=[G.T-R.(K1.(R.q1-X)-K3.(R.q2-Rq1))] J1+G^2.(Jg+Jm) ==
  note: J1+G^2(Jg+Jm).q''
  note: J1+G^2(Jg+Jm)
  note: GT-R(K1(Rq1-X)-K3(Rq2-Rq1)/1/J1+G^2(Jg+Jm)
  Constante 1 : Inport
  "K1 " : Inport  Port=2
  J1 : Inport  Port=3
  G : Inport  Port=4
  Jg : Inport  Port=5
  Jm : Inport  Port=6
  T : Inport  Port=7
  R : Inport  Port=8
  K3 : Inport  Port=9
  q1 : Inport  Port=10
  q2 : Inport  Port=11
  X : Inport  Port=12
  Divide2 : Product  Inputs=*/
  Divide3 : Product  Inputs=*/
  Integrator2 : Integrator
  Product{12..20,22} (10 alike) : Product
  Sum{8..10,12} (4 alike) : Sum  Inputs=|+-
  Sum11 : Sum  Inputs=|++
  Sum13 : Sum  Inputs=|++
  Sum7 : Sum  Inputs=|++
  "TL " : Outport
  wires:
  G/1 -> Product12/1, Product12/2, Product14/1, Divide3/2
  Sum10/1 -> Product19/1  "K1(Rq1-X)-K3(Rq2-Rq1)"
  Product22/1 -> Sum13/1  "q1\""
  Sum8/1 -> Product17/2  "Rq1-X"
  Sum11/1 -> Divide2/2
  "K1 "/1 -> Product17/1
  Product15/1 -> Sum9/2, Sum8/1  "q1*R"
  Divide2/1 -> Product20/1  "1/J1+G^2(Jg+Jm)"
  Product18/1 -> Sum10/2  "K3(Rq2-Rq1)"
  Product13/1 -> Sum11/2  "G^2(Jg+Jm)"
  Product20/1 -> Product22/2, Integrator2/1  "q1\""
  Sum13/1 -> Divide3/1  "GT-R(K1(Rq1-X)-K3(Rq2-Rq1))"
  Product14/1 -> Sum12/1  "G.T"
  Jg/1 -> Sum7/1
  R/1 -> Product19/2, Product15/1, Product16/1
  Product17/1 -> Sum10/1  "K1(Rq1-X)"
  Product16/1 -> Sum9/1  "R.q2"
  Sum12/1 -> Product20/2  "GT-R(K1(Rq1-X)-K3(Rq2-Rq1))"
  Jm/1 -> Sum7/2
  T/1 -> Product14/2
  Sum7/1 -> Product13/2  "Jg+Jm"
  Product19/1 -> Sum13/2, Sum12/2  "R(K1(Rq1-X)-K3(Rq2-Rq1))"
  J1/1 -> Sum11/1
  Sum9/1 -> Product18/1  "Rq1-Rq1"
  K3/1 -> Product18/2
  Product12/1 -> Product13/1  "G^2"
  Constante 1/1 -> Product22/1, Divide2/1
  q1/1 -> Product15/2  "q1"
  q2/1 -> Product16/2  "q1"
  Divide3/1 -> "TL "/1
  X/1 -> Sum8/2  "q1"

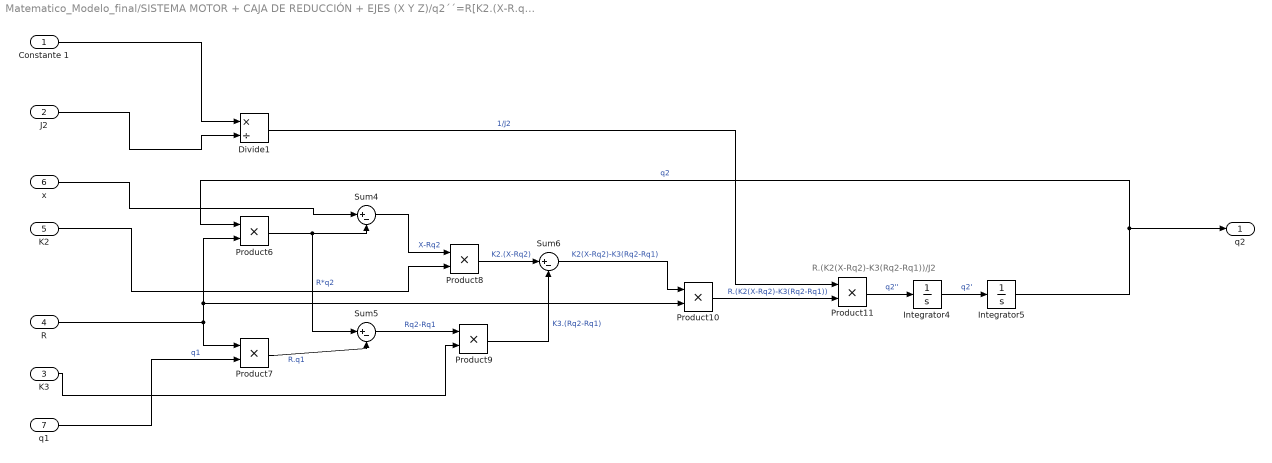
== system Matematico_Modelo_final/SISTEMA MOTOR + CAJA DE REDUCCIÓN + EJES (X Y Z)/q2´´=R[K2.(X-R.q2)-K3.(R.q2-q1)] J2 ==
  note: R.(K2(X-Rq2)-K3(Rq2-Rq1))/J2
  Constante 1 : Inport
  "J2 " : Inport  Port=2
  K3 : Inport  Port=3
  R : Inport  Port=4
  K2 : Inport  Port=5
  x : Inport  Port=6
  q1 : Inport  Port=7
  Divide1 : Product  Inputs=*/
  Integrator4 : Integrator
  Integrator5 : Integrator
  Product{6..11} (6 alike) : Product
  Sum4 : Sum  Inputs=|+-
  Sum5 : Sum  Inputs=|+-
  Sum6 : Sum  Inputs=|+-
  q2 : Outport  VectorParamsAs1DForOutWhenUnconnected=off
  wires:
  Product10/1 -> Product11/2  "R.(K2(X-Rq2)-K3(Rq2-Rq1))"
  Product6/1 -> Sum5/1, Sum4/2  "R*q2"
  Integrator4/1 -> Integrator5/1  "q2'"
  Sum5/1 -> Product9/1  "Rq2-Rq1"
  q1/1 -> Product7/2  "q1"
  Product9/1 -> Sum6/2  "K3.(Rq2-Rq1)"
  "J2 "/1 -> Divide1/2
  Integrator5/1 -> q2/1, Product6/1  "q2"
  Sum4/1 -> Product8/1  "X-Rq2"
  Constante 1/1 -> Divide1/1
  Divide1/1 -> Product11/1  "1/J2"
  R/1 -> Product6/2, Product10/2, Product7/1
  Product7/1 -> Sum5/2  "R.q1"
  K3/1 -> Product9/2
  Product8/1 -> Sum6/1  "K2.(X-Rq2)"
  K2/1 -> Product8/2
  Product11/1 -> Integrator4/1  "q2''"
  Sum6/1 -> Product10/1  "K2(X-Rq2)-K3(Rq2-Rq1)"
  x/1 -> Sum4/1

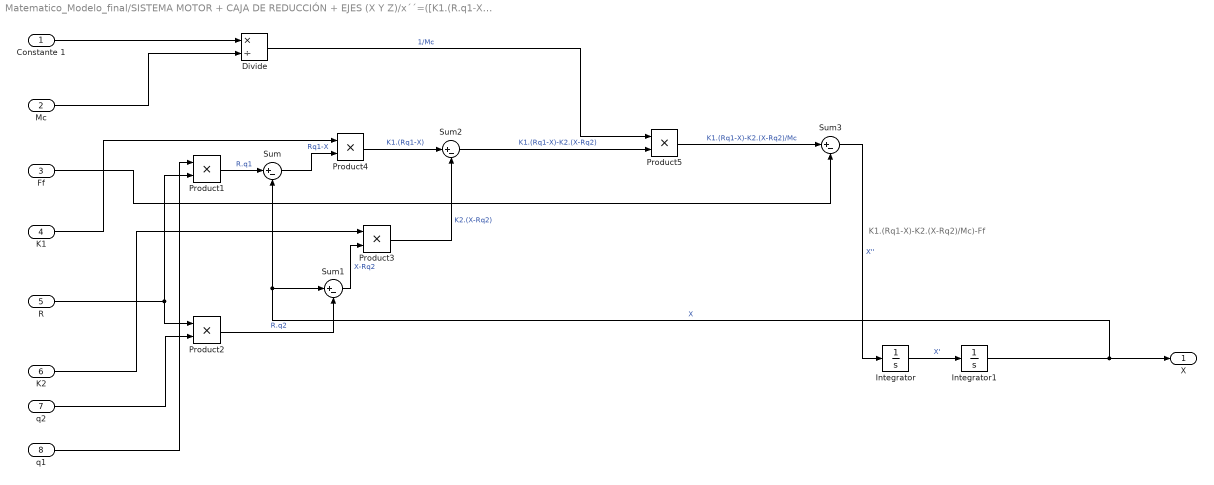
== system Matematico_Modelo_final/SISTEMA MOTOR + CAJA DE REDUCCIÓN + EJES (X Y Z)/x´´=([K1.(R.q1-X)-K2.(X-R.q2)]-Ff) MC ==
  note: K1.(Rq1-X)-K2.(X-Rq2)/Mc)-Ff
  Constante 1 : Inport
  "Mc " : Inport  Port=2
  Ff : Inport  Port=3
  K1 : Inport  Port=4
  R : Inport  Port=5
  K2 : Inport  Port=6
  " q2" : Inport  Port=7
  q1 : Inport  Port=8
  Divide : Product  Inputs=*/
  Integrator : Integrator
  Integrator1 : Integrator
  Product{1..5} (5 alike) : Product
  Sum{,1..3} (4 alike) : Sum  Inputs=|+-
  X : Outport  VectorParamsAs1DForOutWhenUnconnected=off
  wires:
  Sum2/1 -> Product5/2  "K1.(Rq1-X)-K2.(X-Rq2)"
  Sum1/1 -> Product3/2  "X-Rq2"
  Product1/1 -> Sum/1  "R.q1"
  Product4/1 -> Sum2/1  "K1.(Rq1-X)"
  Integrator/1 -> Integrator1/1  "X'"
  Product5/1 -> Sum3/1  "K1.(Rq1-X)-K2.(X-Rq2)/Mc"
  Sum3/1 -> Integrator/1  "X''"
  Divide/1 -> Product5/1  "1/Mc"
  Sum/1 -> Product4/2  "Rq1-X"
  Integrator1/1 -> X/1, Sum/2, Sum1/1  "X"
  Product3/1 -> Sum2/2  "K2.(X-Rq2)"
  Product2/1 -> Sum1/2  "R.q2"
  Constante 1/1 -> Divide/1
  "Mc "/1 -> Divide/2
  Ff/1 -> Sum3/2
  R/1 -> Product1/2, Product2/1
  K2/1 -> Product3/1
  K1/1 -> Product4/1
  " q2"/1 -> Product2/2
  q1/1 -> Product1/1

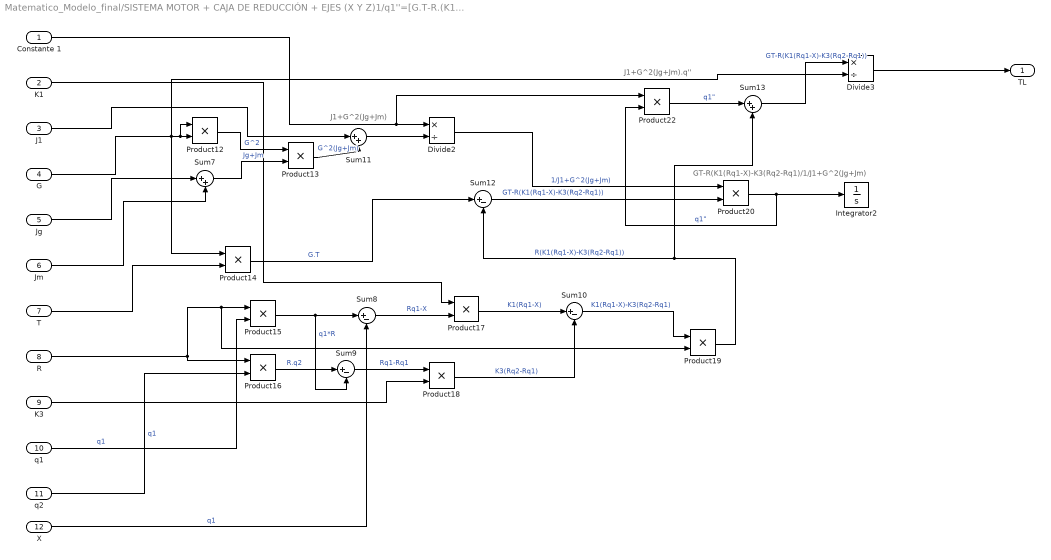
== system Matematico_Modelo_final/SISTEMA MOTOR + CAJA DE REDUCCIÓN + EJES (X Y Z)1/q1''=[G.T-R.(K1.(R.q1-X)-K3.(R.q2-Rq1))] J1+G^2.(Jg+Jm) ==
  note: J1+G^2(Jg+Jm).q''
  note: J1+G^2(Jg+Jm)
  note: GT-R(K1(Rq1-X)-K3(Rq2-Rq1)/1/J1+G^2(Jg+Jm)
  Constante 1 : Inport
  "K1 " : Inport  Port=2
  J1 : Inport  Port=3
  G : Inport  Port=4
  Jg : Inport  Port=5
  Jm : Inport  Port=6
  T : Inport  Port=7
  R : Inport  Port=8
  K3 : Inport  Port=9
  q1 : Inport  Port=10
  q2 : Inport  Port=11
  X : Inport  Port=12
  Divide2 : Product  Inputs=*/
  Divide3 : Product  Inputs=*/
  Integrator2 : Integrator
  Product{12..20,22} (10 alike) : Product
  Sum{8..10,12} (4 alike) : Sum  Inputs=|+-
  Sum11 : Sum  Inputs=|++
  Sum13 : Sum  Inputs=|++
  Sum7 : Sum  Inputs=|++
  "TL " : Outport
  wires:
  G/1 -> Product12/1, Product12/2, Product14/1, Divide3/2
  Sum10/1 -> Product19/1  "K1(Rq1-X)-K3(Rq2-Rq1)"
  Product22/1 -> Sum13/1  "q1\""
  Sum8/1 -> Product17/2  "Rq1-X"
  Sum11/1 -> Divide2/2
  "K1 "/1 -> Product17/1
  Product15/1 -> Sum9/2, Sum8/1  "q1*R"
  Divide2/1 -> Product20/1  "1/J1+G^2(Jg+Jm)"
  Product18/1 -> Sum10/2  "K3(Rq2-Rq1)"
  Product13/1 -> Sum11/2  "G^2(Jg+Jm)"
  Product20/1 -> Product22/2, Integrator2/1  "q1\""
  Sum13/1 -> Divide3/1  "GT-R(K1(Rq1-X)-K3(Rq2-Rq1))"
  Product14/1 -> Sum12/1  "G.T"
  Jg/1 -> Sum7/1
  R/1 -> Product19/2, Product15/1, Product16/1
  Product17/1 -> Sum10/1  "K1(Rq1-X)"
  Product16/1 -> Sum9/1  "R.q2"
  Sum12/1 -> Product20/2  "GT-R(K1(Rq1-X)-K3(Rq2-Rq1))"
  Jm/1 -> Sum7/2
  T/1 -> Product14/2
  Sum7/1 -> Product13/2  "Jg+Jm"
  Product19/1 -> Sum13/2, Sum12/2  "R(K1(Rq1-X)-K3(Rq2-Rq1))"
  J1/1 -> Sum11/1
  Sum9/1 -> Product18/1  "Rq1-Rq1"
  K3/1 -> Product18/2
  Product12/1 -> Product13/1  "G^2"
  Constante 1/1 -> Product22/1, Divide2/1
  q1/1 -> Product15/2  "q1"
  q2/1 -> Product16/2  "q1"
  Divide3/1 -> "TL "/1
  X/1 -> Sum8/2  "q1"

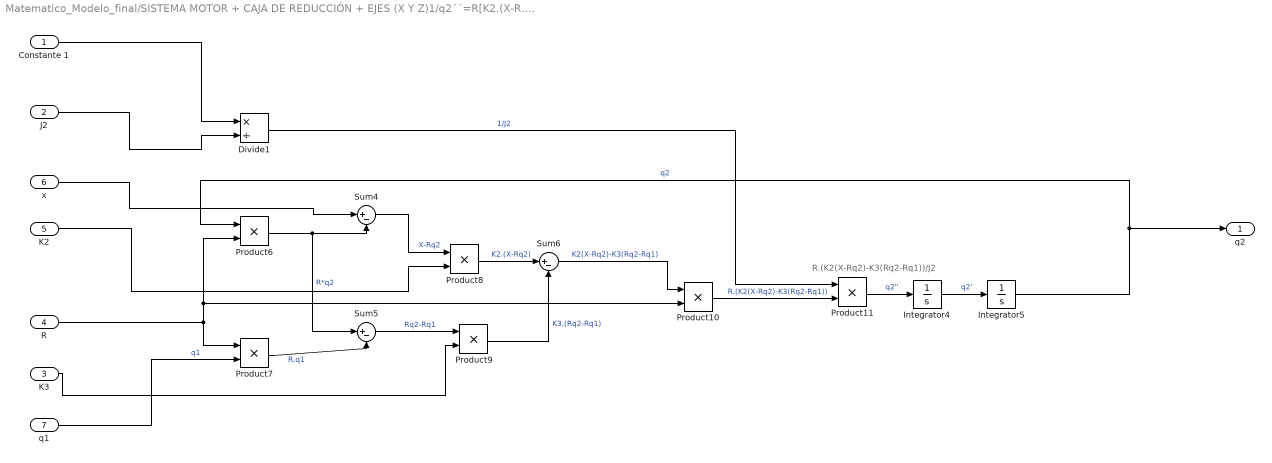
== system Matematico_Modelo_final/SISTEMA MOTOR + CAJA DE REDUCCIÓN + EJES (X Y Z)1/q2´´=R[K2.(X-R.q2)-K3.(R.q2-q1)] J2 ==
  note: R.(K2(X-Rq2)-K3(Rq2-Rq1))/J2
  Constante 1 : Inport
  "J2 " : Inport  Port=2
  K3 : Inport  Port=3
  R : Inport  Port=4
  K2 : Inport  Port=5
  x : Inport  Port=6
  q1 : Inport  Port=7
  Divide1 : Product  Inputs=*/
  Integrator4 : Integrator
  Integrator5 : Integrator
  Product{6..11} (6 alike) : Product
  Sum4 : Sum  Inputs=|+-
  Sum5 : Sum  Inputs=|+-
  Sum6 : Sum  Inputs=|+-
  q2 : Outport  VectorParamsAs1DForOutWhenUnconnected=off
  wires:
  Product10/1 -> Product11/2  "R.(K2(X-Rq2)-K3(Rq2-Rq1))"
  Product6/1 -> Sum5/1, Sum4/2  "R*q2"
  Integrator4/1 -> Integrator5/1  "q2'"
  Sum5/1 -> Product9/1  "Rq2-Rq1"
  q1/1 -> Product7/2  "q1"
  Product9/1 -> Sum6/2  "K3.(Rq2-Rq1)"
  "J2 "/1 -> Divide1/2
  Integrator5/1 -> q2/1, Product6/1  "q2"
  Sum4/1 -> Product8/1  "X-Rq2"
  Constante 1/1 -> Divide1/1
  Divide1/1 -> Product11/1  "1/J2"
  R/1 -> Product6/2, Product10/2, Product7/1
  Product7/1 -> Sum5/2  "R.q1"
  K3/1 -> Product9/2
  Product8/1 -> Sum6/1  "K2.(X-Rq2)"
  K2/1 -> Product8/2
  Product11/1 -> Integrator4/1  "q2''"
  Sum6/1 -> Product10/1  "K2(X-Rq2)-K3(Rq2-Rq1)"
  x/1 -> Sum4/1

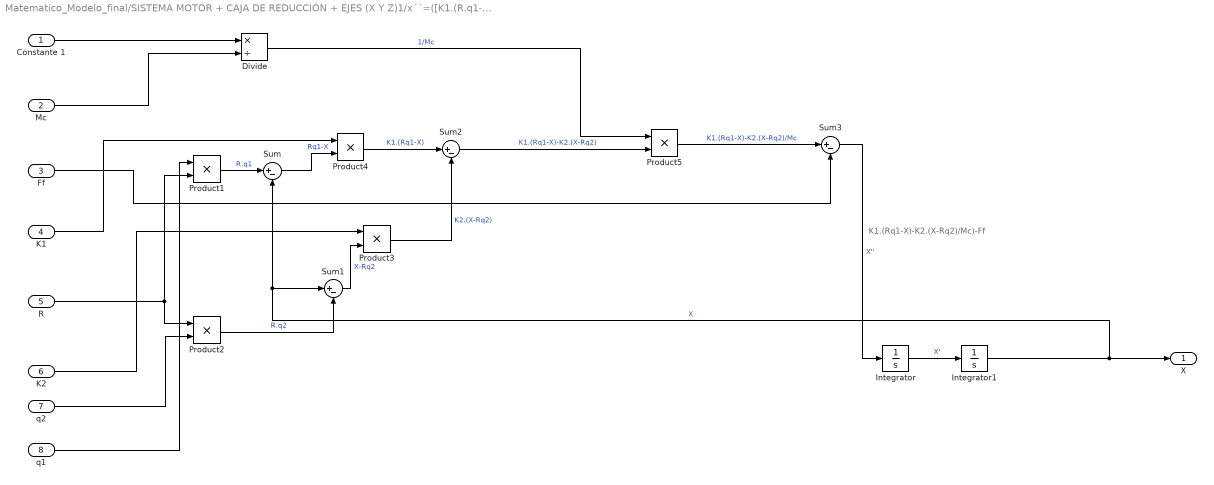
== system Matematico_Modelo_final/SISTEMA MOTOR + CAJA DE REDUCCIÓN + EJES (X Y Z)1/x´´=([K1.(R.q1-X)-K2.(X-R.q2)]-Ff) MC ==
  note: K1.(Rq1-X)-K2.(X-Rq2)/Mc)-Ff
  Constante 1 : Inport
  "Mc " : Inport  Port=2
  Ff : Inport  Port=3
  K1 : Inport  Port=4
  R : Inport  Port=5
  K2 : Inport  Port=6
  " q2" : Inport  Port=7
  q1 : Inport  Port=8
  Divide : Product  Inputs=*/
  Integrator : Integrator
  Integrator1 : Integrator
  Product{1..5} (5 alike) : Product
  Sum{,1..3} (4 alike) : Sum  Inputs=|+-
  X : Outport  VectorParamsAs1DForOutWhenUnconnected=off
  wires:
  Sum2/1 -> Product5/2  "K1.(Rq1-X)-K2.(X-Rq2)"
  Sum1/1 -> Product3/2  "X-Rq2"
  Product1/1 -> Sum/1  "R.q1"
  Product4/1 -> Sum2/1  "K1.(Rq1-X)"
  Integrator/1 -> Integrator1/1  "X'"
  Product5/1 -> Sum3/1  "K1.(Rq1-X)-K2.(X-Rq2)/Mc"
  Sum3/1 -> Integrator/1  "X''"
  Divide/1 -> Product5/1  "1/Mc"
  Sum/1 -> Product4/2  "Rq1-X"
  Integrator1/1 -> X/1, Sum/2, Sum1/1  "X"
  Product3/1 -> Sum2/2  "K2.(X-Rq2)"
  Product2/1 -> Sum1/2  "R.q2"
  Constante 1/1 -> Divide/1
  "Mc "/1 -> Divide/2
  Ff/1 -> Sum3/2
  R/1 -> Product1/2, Product2/1
  K2/1 -> Product3/1
  K1/1 -> Product4/1
  " q2"/1 -> Product2/2
  q1/1 -> Product1/1

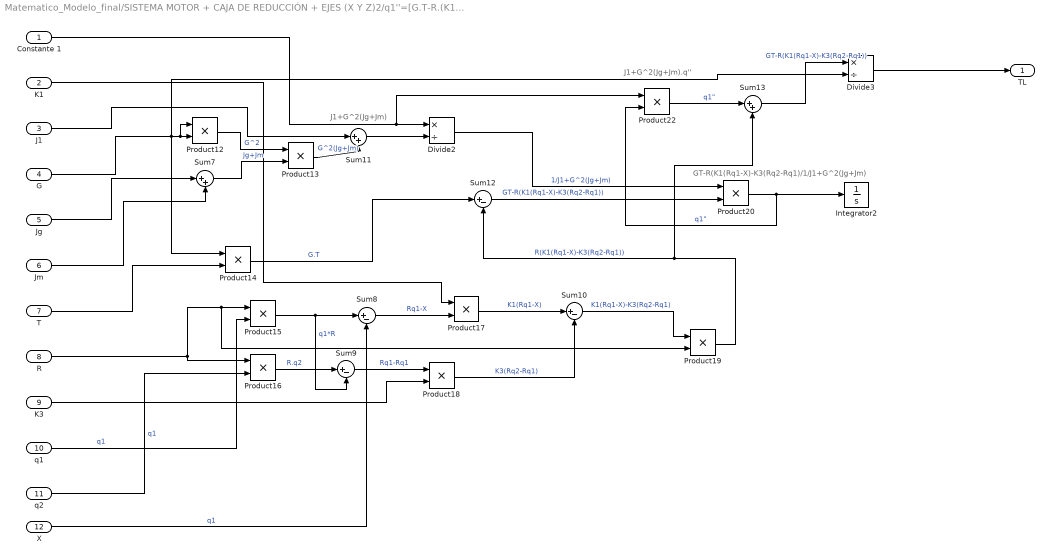
== system Matematico_Modelo_final/SISTEMA MOTOR + CAJA DE REDUCCIÓN + EJES (X Y Z)2/q1''=[G.T-R.(K1.(R.q1-X)-K3.(R.q2-Rq1))] J1+G^2.(Jg+Jm) ==
  note: J1+G^2(Jg+Jm).q''
  note: J1+G^2(Jg+Jm)
  note: GT-R(K1(Rq1-X)-K3(Rq2-Rq1)/1/J1+G^2(Jg+Jm)
  Constante 1 : Inport
  "K1 " : Inport  Port=2
  J1 : Inport  Port=3
  G : Inport  Port=4
  Jg : Inport  Port=5
  Jm : Inport  Port=6
  T : Inport  Port=7
  R : Inport  Port=8
  K3 : Inport  Port=9
  q1 : Inport  Port=10
  q2 : Inport  Port=11
  X : Inport  Port=12
  Divide2 : Product  Inputs=*/
  Divide3 : Product  Inputs=*/
  Integrator2 : Integrator
  Product{12..20,22} (10 alike) : Product
  Sum{8..10,12} (4 alike) : Sum  Inputs=|+-
  Sum11 : Sum  Inputs=|++
  Sum13 : Sum  Inputs=|++
  Sum7 : Sum  Inputs=|++
  "TL " : Outport
  wires:
  G/1 -> Product12/1, Product12/2, Product14/1, Divide3/2
  Sum10/1 -> Product19/1  "K1(Rq1-X)-K3(Rq2-Rq1)"
  Product22/1 -> Sum13/1  "q1\""
  Sum8/1 -> Product17/2  "Rq1-X"
  Sum11/1 -> Divide2/2
  "K1 "/1 -> Product17/1
  Product15/1 -> Sum9/2, Sum8/1  "q1*R"
  Divide2/1 -> Product20/1  "1/J1+G^2(Jg+Jm)"
  Product18/1 -> Sum10/2  "K3(Rq2-Rq1)"
  Product13/1 -> Sum11/2  "G^2(Jg+Jm)"
  Product20/1 -> Product22/2, Integrator2/1  "q1\""
  Sum13/1 -> Divide3/1  "GT-R(K1(Rq1-X)-K3(Rq2-Rq1))"
  Product14/1 -> Sum12/1  "G.T"
  Jg/1 -> Sum7/1
  R/1 -> Product19/2, Product15/1, Product16/1
  Product17/1 -> Sum10/1  "K1(Rq1-X)"
  Product16/1 -> Sum9/1  "R.q2"
  Sum12/1 -> Product20/2  "GT-R(K1(Rq1-X)-K3(Rq2-Rq1))"
  Jm/1 -> Sum7/2
  T/1 -> Product14/2
  Sum7/1 -> Product13/2  "Jg+Jm"
  Product19/1 -> Sum13/2, Sum12/2  "R(K1(Rq1-X)-K3(Rq2-Rq1))"
  J1/1 -> Sum11/1
  Sum9/1 -> Product18/1  "Rq1-Rq1"
  K3/1 -> Product18/2
  Product12/1 -> Product13/1  "G^2"
  Constante 1/1 -> Product22/1, Divide2/1
  q1/1 -> Product15/2  "q1"
  q2/1 -> Product16/2  "q1"
  Divide3/1 -> "TL "/1
  X/1 -> Sum8/2  "q1"

== system Matematico_Modelo_final/SISTEMA MOTOR + CAJA DE REDUCCIÓN + EJES (X Y Z)2/q2´´=R[K2.(X-R.q2)-K3.(R.q2-q1)] J2 ==
  note: R.(K2(X-Rq2)-K3(Rq2-Rq1))/J2
  Constante 1 : Inport
  "J2 " : Inport  Port=2
  K3 : Inport  Port=3
  R : Inport  Port=4
  K2 : Inport  Port=5
  x : Inport  Port=6
  q1 : Inport  Port=7
  Divide1 : Product  Inputs=*/
  Integrator4 : Integrator
  Integrator5 : Integrator
  Product{6..11} (6 alike) : Product
  Sum4 : Sum  Inputs=|+-
  Sum5 : Sum  Inputs=|+-
  Sum6 : Sum  Inputs=|+-
  q2 : Outport  VectorParamsAs1DForOutWhenUnconnected=off
  wires:
  Product10/1 -> Product11/2  "R.(K2(X-Rq2)-K3(Rq2-Rq1))"
  Product6/1 -> Sum5/1, Sum4/2  "R*q2"
  Integrator4/1 -> Integrator5/1  "q2'"
  Sum5/1 -> Product9/1  "Rq2-Rq1"
  q1/1 -> Product7/2  "q1"
  Product9/1 -> Sum6/2  "K3.(Rq2-Rq1)"
  "J2 "/1 -> Divide1/2
  Integrator5/1 -> q2/1, Product6/1  "q2"
  Sum4/1 -> Product8/1  "X-Rq2"
  Constante 1/1 -> Divide1/1
  Divide1/1 -> Product11/1  "1/J2"
  R/1 -> Product6/2, Product10/2, Product7/1
  Product7/1 -> Sum5/2  "R.q1"
  K3/1 -> Product9/2
  Product8/1 -> Sum6/1  "K2.(X-Rq2)"
  K2/1 -> Product8/2
  Product11/1 -> Integrator4/1  "q2''"
  Sum6/1 -> Product10/1  "K2(X-Rq2)-K3(Rq2-Rq1)"
  x/1 -> Sum4/1

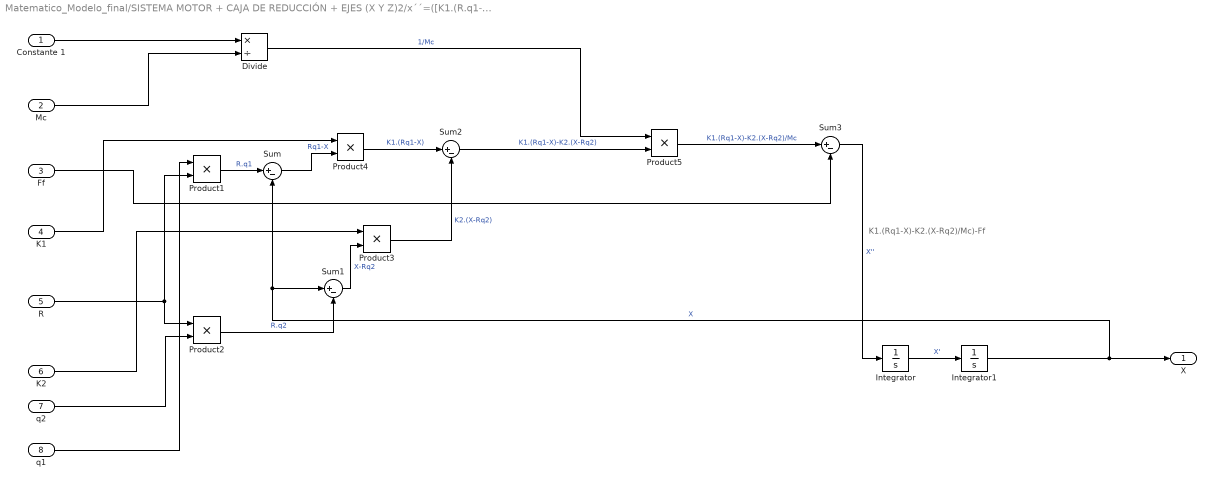
== system Matematico_Modelo_final/SISTEMA MOTOR + CAJA DE REDUCCIÓN + EJES (X Y Z)2/x´´=([K1.(R.q1-X)-K2.(X-R.q2)]-Ff) MC ==
  note: K1.(Rq1-X)-K2.(X-Rq2)/Mc)-Ff
  Constante 1 : Inport
  "Mc " : Inport  Port=2
  Ff : Inport  Port=3
  K1 : Inport  Port=4
  R : Inport  Port=5
  K2 : Inport  Port=6
  " q2" : Inport  Port=7
  q1 : Inport  Port=8
  Divide : Product  Inputs=*/
  Integrator : Integrator
  Integrator1 : Integrator
  Product{1..5} (5 alike) : Product
  Sum{,1..3} (4 alike) : Sum  Inputs=|+-
  X : Outport  VectorParamsAs1DForOutWhenUnconnected=off
  wires:
  Sum2/1 -> Product5/2  "K1.(Rq1-X)-K2.(X-Rq2)"
  Sum1/1 -> Product3/2  "X-Rq2"
  Product1/1 -> Sum/1  "R.q1"
  Product4/1 -> Sum2/1  "K1.(Rq1-X)"
  Integrator/1 -> Integrator1/1  "X'"
  Product5/1 -> Sum3/1  "K1.(Rq1-X)-K2.(X-Rq2)/Mc"
  Sum3/1 -> Integrator/1  "X''"
  Divide/1 -> Product5/1  "1/Mc"
  Sum/1 -> Product4/2  "Rq1-X"
  Integrator1/1 -> X/1, Sum/2, Sum1/1  "X"
  Product3/1 -> Sum2/2  "K2.(X-Rq2)"
  Product2/1 -> Sum1/2  "R.q2"
  Constante 1/1 -> Divide/1
  "Mc "/1 -> Divide/2
  Ff/1 -> Sum3/2
  R/1 -> Product1/2, Product2/1
  K2/1 -> Product3/1
  K1/1 -> Product4/1
  " q2"/1 -> Product2/2
  q1/1 -> Product1/1
